simulink model "circuit_simulation"  (R2021a)
settings: Solver=VariableStepAuto  StartTime=0.0  StopTime=10  RelTol=1e-3
undefined symbols (not defined in the file): C, L, R
settings Model: Creator=Beshary  LastModifiedBy=Beshary
settings DataIOCC: ExternalInput=[t, W]  LoadExternalInput=on

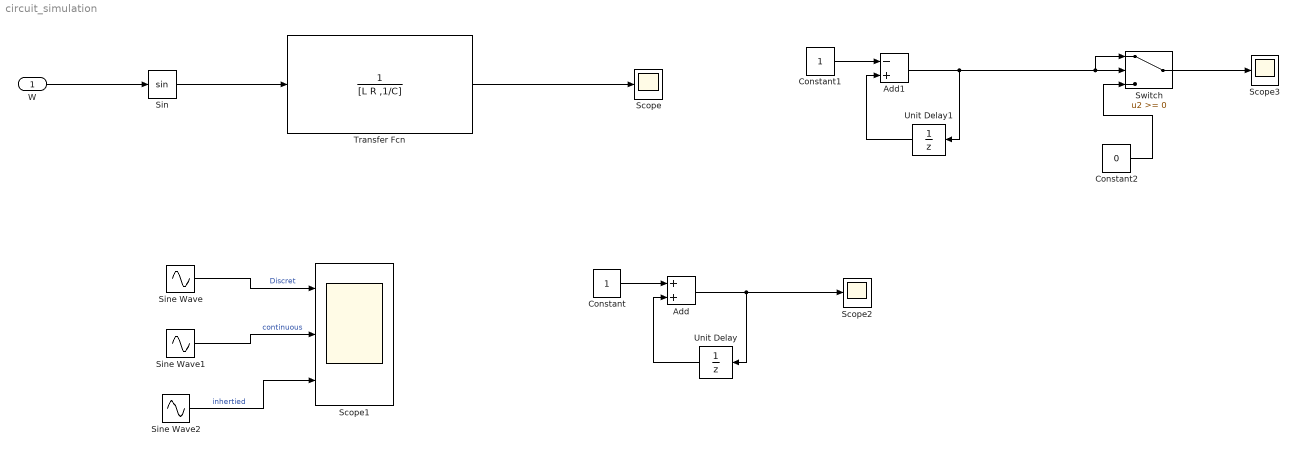
== system circuit_simulation ==
  W : Inport
  Add : Sum
  Add1 : Sum  Inputs=-+
  Constant : Constant
  Constant1 : Constant
  Constant2 : Constant  Value=0
  Scope : Scope
  Scope1 : Scope  NumInputPorts=3
  Scope2 : Scope
  Scope3 : Scope
  Sin : Trigonometry
  Sine Wave : Sin  SampleTime=0.5
  Sine Wave1 : Sin  SampleTime=0
  Sine Wave2 : Sin
  Switch : Switch
  Transfer Fcn : TransferFcn  Numerator=[0 1]  Denominator=[L R ,1/C]
  Unit Delay : UnitDelay  SampleTime=-1  HasFrameUpgradeWarning=on
  Unit Delay1 : UnitDelay  InitialCondition=11  HasFrameUpgradeWarning=on
  wires:
  W/1 -> Sin/1
  Sin/1 -> Transfer Fcn/1
  Transfer Fcn/1 -> Scope/1
  Sine Wave/1 -> Scope1/1  "Discret"
  Sine Wave1/1 -> Scope1/2  "continuous"
  Sine Wave2/1 -> Scope1/3  "inhertied"
  Constant/1 -> Add/1
  Add/1 -> Scope2/1, Unit Delay/1
  Unit Delay/1 -> Add/2
  Constant1/1 -> Add1/1
  Add1/1 -> Switch/1, Switch/2, Unit Delay1/1
  Unit Delay1/1 -> Add1/2
  Switch/1 -> Scope3/1
  Constant2/1 -> Switch/3
